simulink model "sl_rrmc"  (R2022b)
settings: Solver=ode45  StartTime=0.0  StopTime=5.0  RelTol=1e-3  EnableMultiTasking=on
undefined symbols (not defined in the file or in its folder): DiscIntNeverNeededParam
libraries: roblocks x2, visionhdlgeotforms x1
settings Model: Creator=pic  LastModifiedBy=Admin
settings SolverCC: AlgebraicLoopSolver=TrustRegion
settings DataIOCC: SaveFormat=Array  SignalLoggingSaveFormat=ModelDataLogs  SignalLoggingName=sigsOut
settings OptimizationCC: ExpressionDepthLimit=2147483647  LifeSpan=inf
settings DebuggingCC: SaveWithParameterizedLinksMsg=none  UnderspecifiedInitializationDetection=Classic  MergeDetectMultiDrivingBlocksExec=none  SignalResolutionControl=TryResolveAllWithWarning  MultiTaskDSMMsg=warning  MultiTaskCondExecSysMsg=none  FcnCallInpInsideContextMsg=warning  UnconnectedInputMsg=warning  UnconnectedOutputMsg=warning  UnconnectedLineMsg=warning  AllowSymbolicDim=off  StateNameClashWarn=warning  SFUnexpectedBacktrackingDiag=warning  SFNoUnconditionalDefaultTransitionDiag=warning  SFExecutionAtInitializationDiag=none  SFMachineParentedDataDiag=warning  ArithmeticOperatorsInVariantConditions=warning
settings HardwareCC: ProdBitPerPointer=32  ProdBitPerSizeT=32  ProdBitPerPtrDiffT=32  ProdLargestAtomicFloat=None  ProdIntDivRoundTo=Undefined  ProdEndianess=Unspecified  ProdWordSize=32  ProdHWDeviceType=32-bit Generic  TargetUnknown=on
settings ModelReferenceCC: EnableRefExpFcnMdlSchedulingChecks=on  PropagateSignalLabelsOutOfModel=off
settings SFSimCC: SimUseLocalCustomCode=off  CustomCodeUndefinedFunction=UseInterfaceOnly
settings RTWCC: RTWUseLocalCustomCode=off
settings CodeAppCC: StateflowObjectComments=on
settings GRTTargetCC: TargetLangStandard=C89/C90 (ANSI)  CombineOutputUpdateFcns=off  GRTInterface=on
settings ConfigComp: CovMetricSettings=dw  CovSaveCumulativeToWorkspaceVar=on  CovSaveSingleToWorkspaceVar=on  CovExternalEMLEnable=off

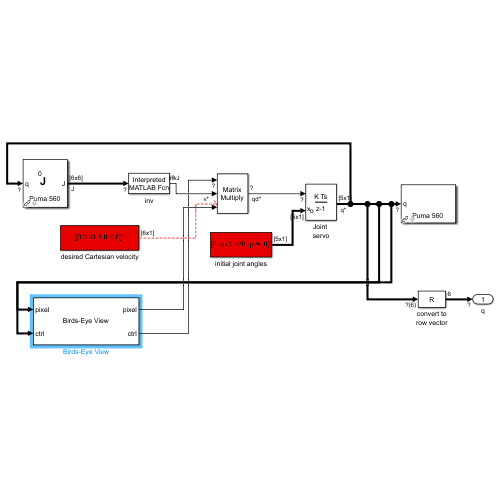
[thumbnail: Simulink's stored preview of the top-level diagram]
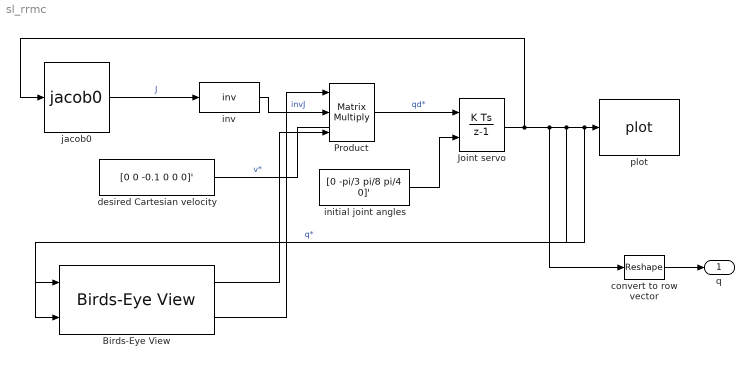
== system sl_rrmc ==
  Birds-Eye View : visionhdlgeotforms/Birds-Eye View  HomographyMatrix=[0.000100990123328 0 0;0.000412396945637 0.001302203393162 1.293171994e-06;-0.103019798961327 -0.255811259450009 -0.000222053779501]  MaxBufferSize=40000  MaxSourceLinesBuffered=54  BirdsEyeActivePixels=640  BirdsEyeActiveLines=700  SimulateUsing=Code generation
  Joint servo : DiscreteIntegrator  InitialConditionSource=external  InitialCondition=[0 pi/4 pi 0 pi/4 0]'  SampleTime=0.05  ICPrevOutput=DiscIntNeverNeededParam  ICPrevScaledInput=DiscIntNeverNeededParam
  Product : Product  Inputs=3  Multiplication=Matrix(*)  SaturateOnIntegerOverflow=on  OutDataTypeStr=Inherit: Same as first input
  convert to row vector : Reshape  OutputDimensionality=Customize  OutputDimensions=6
  desired Cartesian velocity : Constant  Value=[0 0 -0.1 0 0 0]'  VectorParams1D=off
  initial joint angles : Constant  Value="[0 -pi/3 pi/8  pi/4 0]'"  VectorParams1D=off
  inv : MATLABFcn  MATLABFcn=inv  Output1D=off
  "jacob0 " : roblocks/Arm/jacob0   robot=p560
  plot : roblocks/Arm/plot  robot=p560  fps=25  holdplot=on
  q : Outport
  wires:
  "jacob0 "/1 -> inv/1  "J"
  Joint servo/1 -> Birds-Eye View/2, Birds-Eye View/1, plot/1, convert to row vector/1, "jacob0 "/1  "q*"
  inv/1 -> Product/2  "invJ"
  desired Cartesian velocity/1 -> ?  "v*"
  convert to row vector/1 -> q/1
  Product/1 -> Joint servo/1  "qd*"
  initial joint angles/1 -> Joint servo/2
  Birds-Eye View/1 -> Product/3
  Birds-Eye View/2 -> Product/1
